simulink model "omni_server"  (Simulink 7.0)
settings: Solver=ode1  StartTime=0.0  StopTime=inf  FixedStep=0.001  RelTol=1e-3
libraries: quarc_library x3
settings Model: Creator=colinlea  LastModifiedBy=colinlea  SimulationMode=external  ExtModeTrigDuration=10000
settings SolverCC: PositivePriorityOrder=on
settings RTWCC: SystemTargetFile=quarc_windows.tlc  TemplateMakefile=quarc_default_tmf  Description=QuaRC Win32 Target  ProcessScript=quarc_windows_make_rtw_hook
settings STFCustomTargetCC: TargetPreCompLibLocation=C:\DOCUME~1\ALLUSE~1\APPLIC~1\QuaRC\lib\2007b\windows\release  GenFloatMathFcnCalls=ANSI_C  SystemTargetFile=quarc_windows.tlc
settings GRTTargetCC: TargetPreCompLibLocation=C:\DOCUME~1\ALLUSE~1\APPLIC~1\QuaRC\lib\2007b\windows\release  CompOptLevelCompliant=off  MatFileLogging=off  ExtMode=on  ExtModeMexFile=quarc_comm

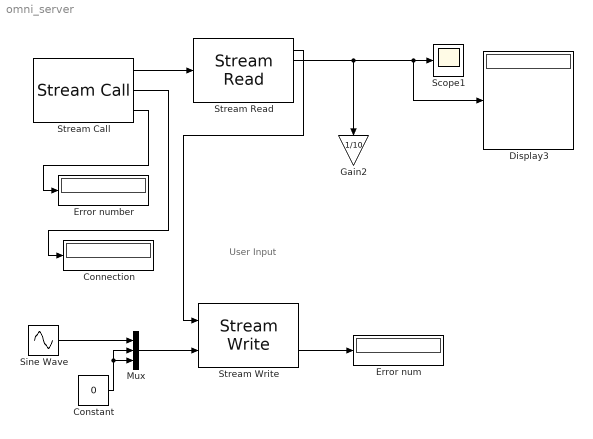
== system omni_server ==
  note: User Input
  Connection : Display
  Constant : Constant  Value=0  OutDataType=sfix(16)  OutScaling=2^0
  Display3 : Display
  Error num : Display
  Error number : Display
  Gain2 : Gain  Orientation=down  Gain=1/10  ParameterDataType=sfix(16)  ParameterScaling=2^0  OutDataType=sfix(16)  OutScaling=2^0
  Mux : Mux  Inputs=3
  Scope1 : Scope
      settings: YMin=-1  YMax=1
  Sine Wave : Sin  Amplitude=.2  Frequency=20  SampleTime=0
  Stream Call : quarc_library/Communications/Intermediate/Stream Call  uri_source=Internal (dialog parameter)  uri=tcpip://localhost:18000  send_buffer_size=8000  receive_buffer_size=8000  byte_order=little endian (Intel - LSB first)  sample_time=qc_get_step_size  active=off
      settings: AttributesFormatString=(%<uri>)
  Stream Read : quarc_library/Communications/Intermediate/Stream Read  data_type=Inherited via back propagation  num_elements=3
  Stream Write : quarc_library/Communications/Intermediate/Stream Write  optimization=Minimizing latency
  wires:
  Stream Call/1 -> Stream Read/1
  Stream Read/2 -> Scope1/1, Display3/1, Gain2/1
  Stream Call/2 -> Connection/1
  Stream Call/3 -> Error number/1
  Sine Wave/1 -> Mux/1
  Constant/1 -> Mux/2, Mux/3
  Mux/1 -> Stream Write/2
  Stream Write/2 -> Error num/1
  Stream Read/1 -> Stream Write/1
